simulink model "kadai11"  (R2021b)
settings: Solver=VariableStepAuto  StartTime=0.0  StopTime=10.0  RelTol=1e-3
settings Model: Creator=is221042  LastModifiedBy=is221042

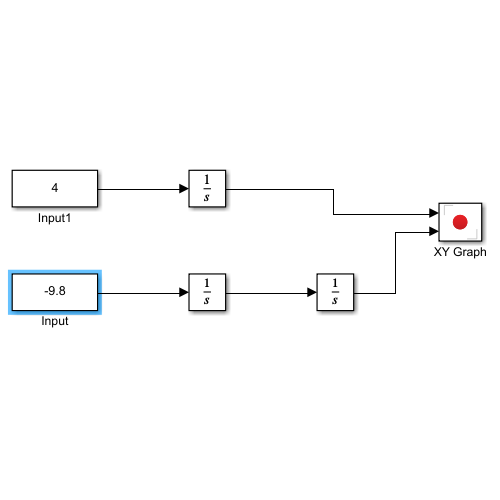
[thumbnail: Simulink's stored preview of the top-level diagram]
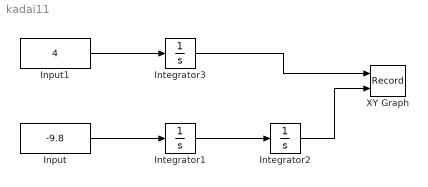
== system kadai11 ==
  Input : Constant  Value=-9.8
  Input1 : Constant  Value=4
  Integrator1 : Integrator
  Integrator2 : Integrator
  Integrator3 : Integrator
  XY Graph : Record  FileSettingsInternal="{\"entries\":[{\"content\":{\"excelSettings\":{\"content\":{},\"type\":\"Streamout.ExcelSettings\"}},\"type\":\"Streamout.FileSettingStorage\",\"uuid\":\"c8e75054-5216-47d1-a5a3-b5ef42cb6580\"}],\"packageUris\":[\"http://schema.mathworks.com/mf0/streamout_blocks/R2020a\"],\"version\":\"1.0\"}"  Layout=[1 1]  SignalsInternal="{\"entries\":[{\"content\":{\"signals\":[{\"content\":{\"blockPath\":[\"untitled/XY Graph\"],\"channel\":[],\"dimensions\":[1],\"domain\":\"untitled/XY Graph\",\"lineColor\":\"#a2142f\",\"plots\":[1],\"port\":1,\"sid\":[\"\"],\"signalID\":28,\"signalName\":\"Integrator3\"},\"type\":\"RecordBlkView.Signal\",\"uuid\":\"c5acacee-5058-47a5-a060-b4fa287ea74c\"},{\"content\":{\"blockPath\":[\"untitled/XY Graph\"],\"channel\":[],\"dimensions\":[1],\"domain\":\"untitled/XY Graph\",\"lineColor\":\"#139fff\",\"plots\":[1],\"port\":2,\"sid\":[\"\"],\"signalID\":32,\"signalName\":\"Integrator2\"},\"type\":\"RecordBlkView.Signal\",\"uuid\":\"244915fc-cb33-439d-89f6-346157684e22\"}]},\"type\":\"RecordBlkView.InputSignals\",\"uuid\":\"495ac2f0-10df-46a3-9b3c-31f4426ce8cd\"}],\"packageUris\":[\"http://schema.mathworks.com/mf0/streamout_blocks/R2020a\"],\"version\":\"1.0\"}"  VisualizationBindings="{\"xyplotplugin\":{\"info\":[{\"series\":[{\"bindingParametersList\":[{\"parameter\":\"X-Axis\",\"signalID\":28,\"signalName\":\"Integrator3\"},{\"parameter\":\"Y-Axis\",\"signalID\":32,\"signalName\":\"Integrator2\"}],\"seriesID\":5642}],\"subplotID\":1}]}}"  CompatibilityTag=XY
  wires:
  Integrator3/1 -> XY Graph/1
  Integrator2/1 -> XY Graph/2
  Integrator1/1 -> Integrator2/1
  Input1/1 -> Integrator3/1
  Input/1 -> Integrator1/1
